simulink model "DCDCConverter"  (R2021a)
settings: Solver=VariableStepAuto  StartTime=0.0  StopTime=10.0  RelTol=1e-3
libraries: spsIdealSwitchLib x4, spsSeriesRLCBranchLib x2, spsDiodeLib x2, spsVoltageMeasurementLib x2, spsDCVoltageSourceLib x1, spsLinearTransformerLib x1, spspowerguiLib x1
settings Model: Creator=msipc  LastModifiedBy=msipc

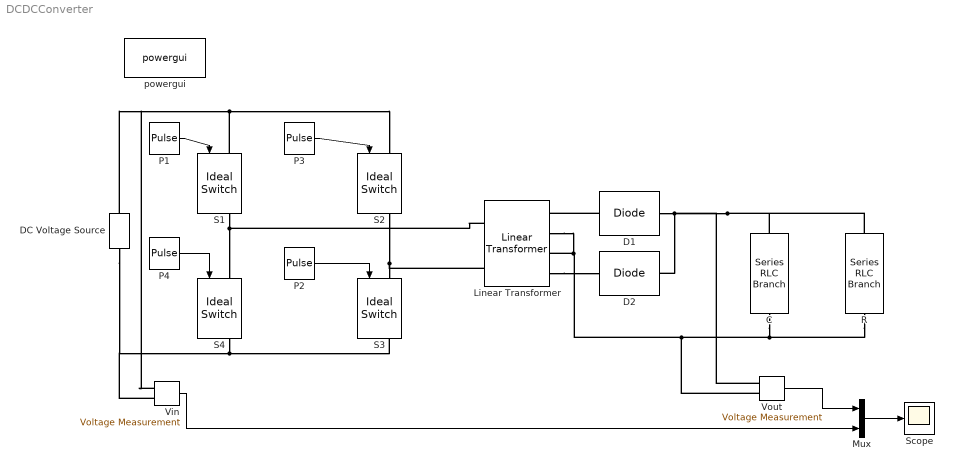
== system DCDCConverter ==
  C : spsSeriesRLCBranchLib/Series RLC Branch  LConnTagsString=__new0  RConnTagsString=__new0  BranchType=RLC  Resistance=1  Inductance=1e-3  SetiL0=off  InitialCurrent=0  Capacitance=100e-6  Setx0=off  InitialVoltage=0  Measurements=None
  "D1\t" : spsDiodeLib/Diode  Ron=0.001  Lon=0  Vf=0.8  IC=0  UseSnubber=0  Rs=1e12  Cs=inf  Measurements=off
  D2 : spsDiodeLib/Diode  Ron=0.001  Lon=0  Vf=0.8  IC=0  UseSnubber=0  Rs=1e12  Cs=inf  Measurements=off
  DC Voltage Source : spsDCVoltageSourceLib/DC Voltage Source  Amplitude=46.8  Measurements=None
  Linear Transformer : spsLinearTransformerLib/Linear Transformer  UNITS=pu  NominalPower=[ 50 50 ]  winding1="[ 46.8/1.4142  0.002  0.0005 ]"  winding2="[ 46.8/1.4142  0.002  0.0005 ]"  ThreeWindings=on  winding3="[ 46.8/1.4142  0.002  0.0005 ]"  RmLm=[ 500 500 ]  Measurements=None  DataType=off
  Mux : Mux  Inputs=2
  P1 : DiscretePulseGenerator  PulseType=Time based  Period=10  PulseWidth=0.02
  P2 : DiscretePulseGenerator  PulseType=Time based  Period=10  PulseWidth=0.02
  P3 : DiscretePulseGenerator  PulseType=Time based  Period=10  PulseWidth=0.02  PhaseDelay=180*0.02/360
  P4 : DiscretePulseGenerator  PulseType=Time based  Period=10  PulseWidth=0.02  PhaseDelay=180*0.02/360
  R : spsSeriesRLCBranchLib/Series RLC Branch  LConnTagsString=__new0  RConnTagsString=__new0  BranchType=RLC  Resistance=10  Inductance=1e-3  SetiL0=off  InitialCurrent=0  Capacitance=1e-6  Setx0=off  InitialVoltage=0  Measurements=None
  S{1..4} (4 alike) : spsIdealSwitchLib/Ideal Switch  Ron=0.001  Lon=0  IC=0  Rs=1e5  Cs=inf  Measurements=on
  Scope : Scope
  Vin : spsVoltageMeasurementLib/Voltage Measurement  PhasorSimulation=off  OutputType=Complex  PSBequivalent=0
  Vout : spsVoltageMeasurementLib/Voltage Measurement  PhasorSimulation=off  OutputType=Complex  PSBequivalent=0
  powergui : spspowerguiLib/powergui  Priority=1  SimulationMode=Discrete  SampleTime=50e-6  frequency=60  Iterations=50  frequencyindice=0  Pbase=100e6  ErrMax=1e-4  UnitsV=kV  UnitsW=MW  buscounter=0  FunctionMessages=off  echomessages=off  EnableUseOfTLC=off  CurrentSourceSwitches=off  DisableSnubberDevices=off  DisableRonSwitches=off  DisableVfSwitches=off  DisplayEquations=off  AutomaticDiscreteSolvers=off  SolverType=Tustin/Backward Euler (TBE)  Interpol=off  ExternalGateDelay=off  methode=off  Ts=100  x0status=blocks  SPID=on  SwTol=0  HookPort=off  NonlinearTolerance=1e-4  nMaxIteration=100  ContinueOnMaxIteration=off  RestoreLinks=warning  ResistiveCurrentMeasurement=off  Frange=[0:2:500]  Ylog=off  Xlog=on  ShowGrid=off  save=off  variable=ZData  structure=0  ZoomFFT=off  StartTime=0.0  cycles=1  DisplayStyle=1  fundamental=60  FreqAxis=off  MaxFrequency=1000  frequencyindicesteady=1  RmsSteady=1  display=off
  wires:
  P1/1 -> S1/1
  P2/1 -> S3/1
  P3/1 -> S2/1
  P4/1 -> S4/1
  Vout/1 -> Mux/1
  Vin/1 -> Mux/2
  Mux/1 -> Scope/1
  connections:
  S1/LConn1 -- Vin/LConn1 -- DC Voltage Source/RConn1 -- S2/LConn1
  S2/RConn1 -- Linear Transformer/LConn2 -- S3/LConn1
  S1/RConn1 -- S4/LConn1 -- Linear Transformer/LConn1
  S4/RConn1 -- Vin/LConn2 -- DC Voltage Source/LConn1 -- S3/RConn1
  "D1\t"/LConn1 -- Linear Transformer/RConn1
  Linear Transformer/RConn4 -- D2/LConn1
  "D1\t"/RConn1 -- R/LConn1 -- C/LConn1 -- Vout/LConn1 -- D2/RConn1
  C/RConn1 -- R/RConn1 -- Vout/LConn2 -- Linear Transformer/RConn2 -- Linear Transformer/RConn3
